simulink model "MultipleAgentsChoice_NoVR"  (R2013b)
settings: Solver=ode45  StartTime=0.0  StopTime=1000  RelTol=1e-4  AbsTol=1e-4
libraries: simulink x24
(part 4 of 5)

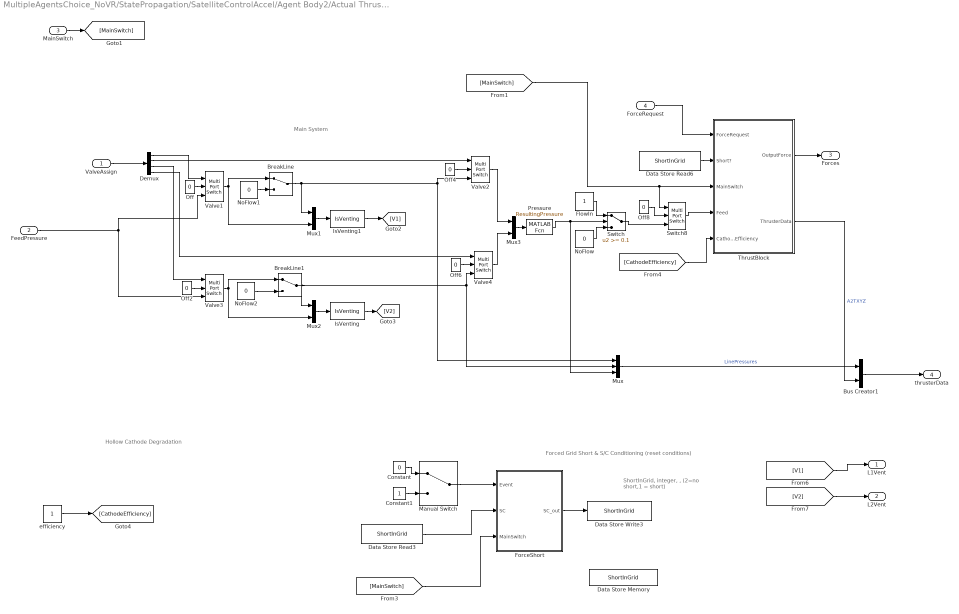
== system MultipleAgentsChoice_NoVR/StatePropagation/SatelliteControlAccel/Agent Body2/Actual Thruster response/XYZthruster/Thruster1 ==
  note: Main System
  note: Hollow Cathode Degradation
  note: ShortInGrid, integer, , (2=no short,1 = short)
  note: Forced Grid Short & S/C Conditioning (reset conditions)
  ValveAssign : Inport
  FeedPressure : Inport  Port=2
  MainSwitch : Inport  Port=3
  ForceRequest : Inport  Port=4
  BreakLine : ManualSwitch
  BreakLine1 : ManualSwitch
  Bus Creator1 : BusCreator  Inputs=2
  Constant : Constant  Value=0
  Constant1 : Constant
  Data Store Memory : DataStoreMemory  DataStoreName=ShortInGrid  ReadBeforeWriteMsg=warning  WriteAfterWriteMsg=warning  WriteAfterReadMsg=warning  InitialValue=2
  Data Store Read3 : DataStoreRead  DataStoreName=ShortInGrid  SampleTime=0
  Data Store Read6 : DataStoreRead  DataStoreName=ShortInGrid  SampleTime=0
  Data Store Write3 : DataStoreWrite  DataStoreName=ShortInGrid
  Demux : Demux
  FlowIn : Constant
  ForceShort : Subsystem
  IsVenting : MATLABFcn  MATLABFcn=IsVenting  OutputDimensions=1
  IsVenting1 : MATLABFcn  MATLABFcn=IsVenting  OutputDimensions=1
  Manual Switch : ManualSwitch
  Mux : Mux  Inputs=3
  Mux1 : Mux  Inputs=2
  Mux2 : Mux  Inputs=2
  Mux3 : Mux  Inputs=2
  NoFlow : Constant  Value=0
  NoFlow1 : Constant  Value=0
  NoFlow2 : Constant  Value=0
  Off{,2,4,6,8} (5 alike) : Constant  Value=0
  Pressure : MATLABFcn  MATLABFcn=ResultingPressure
  Switch : Switch  Threshold=0.1
  Switch8 : MultiPortSwitch  Inputs=2
  ThrustBlock : Subsystem
  Valve{1..4} (4 alike) : MultiPortSwitch  Inputs=2
  efficiency : Constant
  L1Vent : Outport
  L2Vent : Outport  Port=2
  Forces : Outport  Port=3
  thrusterData : Outport  Port=4
  wires:
  [MainSwitch] -> Switch8/1, ThrustBlock/3(MainSwitch)
  Valve4/1 -> Mux3/2
  MainSwitch/1 -> [MainSwitch]
  FeedPressure/1 -> Valve3/3, Valve1/3
  IsVenting/1 -> [V2]
  IsVenting1/1 -> [V1]
  Pressure/1 -> Mux/3, Switch/2
  Mux2/1 -> IsVenting/1
  Mux1/1 -> IsVenting1/1
  Bus Creator1/1 -> thrusterData/1
  ForceRequest/1 -> ThrustBlock/1(ForceRequest)
  [CathodeEfficiency] -> ThrustBlock/5(CathodeEfficiency)
  BreakLine1/1 -> Mux/2, Valve4/3, Mux2/1
  Valve3/1 -> Mux2/2, BreakLine1/1
  NoFlow2/1 -> BreakLine1/2
  Mux/1 -> Bus Creator1/1  "LinePressures"
  Switch/1 -> Switch8/3
  Off8/1 -> Switch8/2
  Off6/1 -> Valve4/2
  Off2/1 -> Valve3/2
  Off4/1 -> Valve2/2
  Off/1 -> Valve1/2
  NoFlow1/1 -> BreakLine/2
  ThrustBlock/1(OutputForce) -> Forces/1
  ThrustBlock/2(ThrusterData) -> Bus Creator1/2  "A2TXYZ"
  Demux/4 -> Valve4/1
  Demux/3 -> Valve3/1
  Demux/2 -> Valve2/1
  Demux/1 -> Valve1/1
  ValveAssign/1 -> Demux/1
  Data Store Read6/1 -> ThrustBlock/2(Short?)
  Switch8/1 -> ThrustBlock/4(Feed)
  NoFlow/1 -> Switch/3
  FlowIn/1 -> Switch/1
  BreakLine/1 -> Mux/1, Valve2/3, Mux1/1
  Mux3/1 -> Pressure/1
  Valve2/1 -> Mux3/1
  Valve1/1 -> Mux1/2, BreakLine/1
  efficiency/1 -> [CathodeEfficiency]
  [MainSwitch] -> ForceShort/3(MainSwitch)
  Data Store Read3/1 -> ForceShort/2(SC)
  Manual Switch/1 -> ForceShort/1(Event)
  Constant1/1 -> Manual Switch/2
  Constant/1 -> Manual Switch/1
  ForceShort/1(SC_out) -> Data Store Write3/1
  [V1] -> L1Vent/1
  [V2] -> L2Vent/1

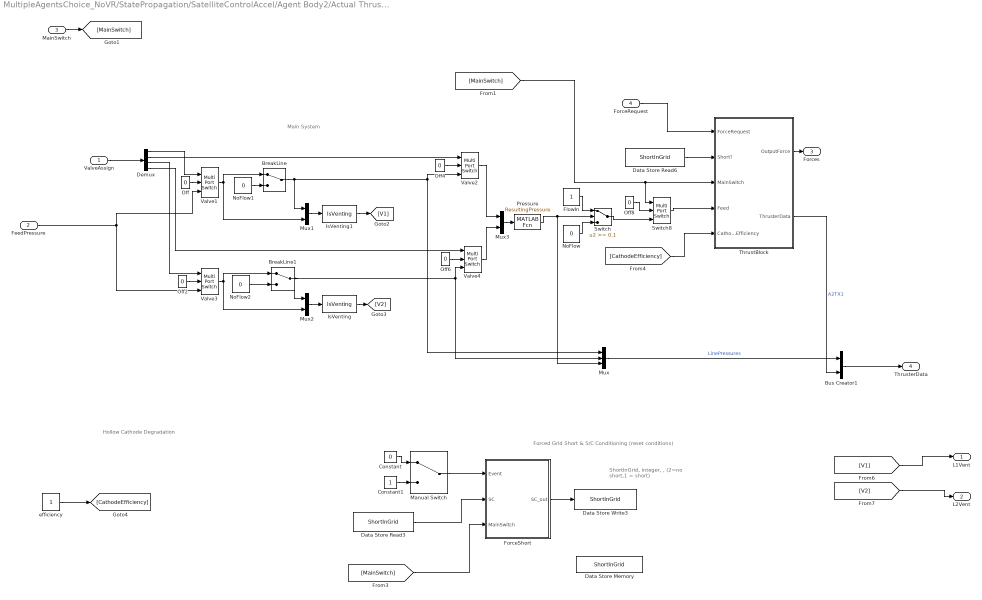
== system MultipleAgentsChoice_NoVR/StatePropagation/SatelliteControlAccel/Agent Body2/Actual Thruster response/Xthruster/Thruster1 ==
  note: Forced Grid Short & S/C Conditioning (reset conditions)
  note: ShortInGrid, integer, , (2=no short,1 = short)
  note: Hollow Cathode Degradation
  note: Main System
  ValveAssign : Inport
  FeedPressure : Inport  Port=2
  MainSwitch : Inport  Port=3
  ForceRequest : Inport  Port=4
  BreakLine : ManualSwitch
  BreakLine1 : ManualSwitch
  Bus Creator1 : BusCreator  Inputs=2
  Constant : Constant  Value=0
  Constant1 : Constant
  Data Store Memory : DataStoreMemory  DataStoreName=ShortInGrid  ReadBeforeWriteMsg=warning  WriteAfterWriteMsg=warning  WriteAfterReadMsg=warning  InitialValue=2
  Data Store Read3 : DataStoreRead  DataStoreName=ShortInGrid  SampleTime=0
  Data Store Read6 : DataStoreRead  DataStoreName=ShortInGrid  SampleTime=0
  Data Store Write3 : DataStoreWrite  DataStoreName=ShortInGrid
  Demux : Demux
  FlowIn : Constant
  ForceShort : Subsystem
  IsVenting : MATLABFcn  MATLABFcn=IsVenting  OutputDimensions=1
  IsVenting1 : MATLABFcn  MATLABFcn=IsVenting  OutputDimensions=1
  Manual Switch : ManualSwitch
  Mux : Mux  Inputs=3
  Mux1 : Mux  Inputs=2
  Mux2 : Mux  Inputs=2
  Mux3 : Mux  Inputs=2
  NoFlow : Constant  Value=0
  NoFlow1 : Constant  Value=0
  NoFlow2 : Constant  Value=0
  Off{,2,4,6,8} (5 alike) : Constant  Value=0
  Pressure : MATLABFcn  MATLABFcn=ResultingPressure
  Switch : Switch  Threshold=0.1
  Switch8 : MultiPortSwitch  Inputs=2
  ThrustBlock : Subsystem
  Valve{1..4} (4 alike) : MultiPortSwitch  Inputs=2
  efficiency : Constant
  L1Vent : Outport
  L2Vent : Outport  Port=2
  Forces : Outport  Port=3
  ThrusterData : Outport  Port=4
  wires:
  ForceShort/1(SC_out) -> Data Store Write3/1
  Constant/1 -> Manual Switch/1
  Constant1/1 -> Manual Switch/2
  Manual Switch/1 -> ForceShort/1(Event)
  Data Store Read3/1 -> ForceShort/2(SC)
  [MainSwitch] -> ForceShort/3(MainSwitch)
  efficiency/1 -> [CathodeEfficiency]
  Valve1/1 -> BreakLine/1, Mux1/2
  Valve2/1 -> Mux3/1
  Mux3/1 -> Pressure/1
  BreakLine/1 -> Mux1/1, Valve2/3, Mux/1
  FlowIn/1 -> Switch/1
  NoFlow/1 -> Switch/3
  Switch8/1 -> ThrustBlock/4(Feed)
  Data Store Read6/1 -> ThrustBlock/2(Short?)
  ValveAssign/1 -> Demux/1
  Demux/1 -> Valve1/1
  Demux/2 -> Valve2/1
  Demux/3 -> Valve3/1
  Demux/4 -> Valve4/1
  ThrustBlock/2(ThrusterData) -> Bus Creator1/2  "A2TX1"
  ThrustBlock/1(OutputForce) -> Forces/1
  NoFlow1/1 -> BreakLine/2
  Off/1 -> Valve1/2
  Off4/1 -> Valve2/2
  Off2/1 -> Valve3/2
  Off6/1 -> Valve4/2
  Off8/1 -> Switch8/2
  Switch/1 -> Switch8/3
  Mux/1 -> Bus Creator1/1  "LinePressures"
  NoFlow2/1 -> BreakLine1/2
  Valve3/1 -> BreakLine1/1, Mux2/2
  BreakLine1/1 -> Mux2/1, Valve4/3, Mux/2
  [CathodeEfficiency] -> ThrustBlock/5(CathodeEfficiency)
  ForceRequest/1 -> ThrustBlock/1(ForceRequest)
  Bus Creator1/1 -> ThrusterData/1
  Mux1/1 -> IsVenting1/1
  Mux2/1 -> IsVenting/1
  Pressure/1 -> Switch/2, Mux/3
  IsVenting1/1 -> [V1]
  IsVenting/1 -> [V2]
  FeedPressure/1 -> Valve1/3, Valve3/3
  MainSwitch/1 -> [MainSwitch]
  Valve4/1 -> Mux3/2
  [MainSwitch] -> ThrustBlock/3(MainSwitch), Switch8/1
  [V1] -> L1Vent/1
  [V2] -> L2Vent/1

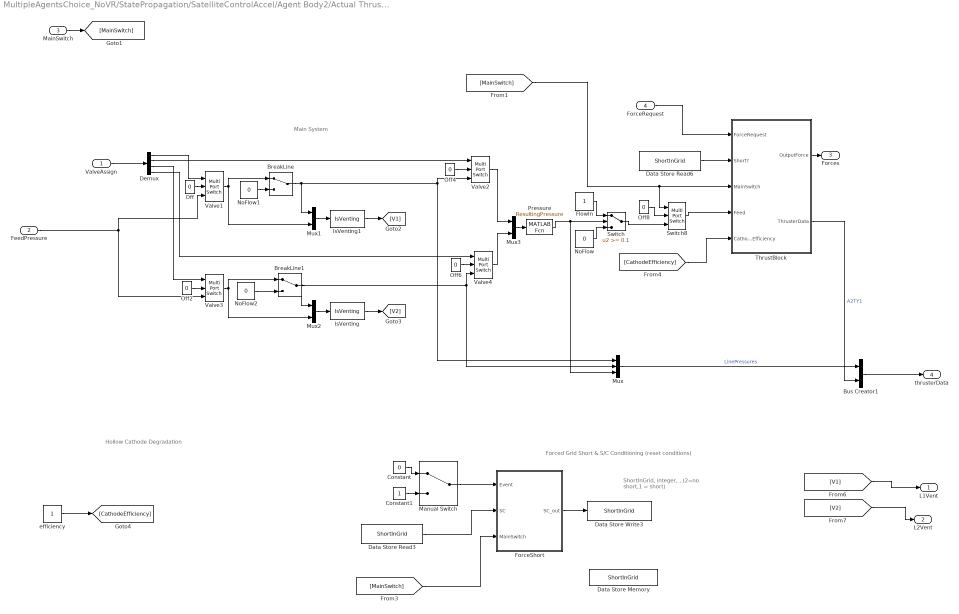
== system MultipleAgentsChoice_NoVR/StatePropagation/SatelliteControlAccel/Agent Body2/Actual Thruster response/Ythruster1/Thruster1 ==
  note: Main System
  note: Hollow Cathode Degradation
  note: ShortInGrid, integer, , (2=no short,1 = short)
  note: Forced Grid Short & S/C Conditioning (reset conditions)
  ValveAssign : Inport
  FeedPressure : Inport  Port=2
  MainSwitch : Inport  Port=3
  ForceRequest : Inport  Port=4
  BreakLine : ManualSwitch
  BreakLine1 : ManualSwitch
  Bus Creator1 : BusCreator  Inputs=2
  Constant : Constant  Value=0
  Constant1 : Constant
  Data Store Memory : DataStoreMemory  DataStoreName=ShortInGrid  ReadBeforeWriteMsg=warning  WriteAfterWriteMsg=warning  WriteAfterReadMsg=warning  InitialValue=2
  Data Store Read3 : DataStoreRead  DataStoreName=ShortInGrid  SampleTime=0
  Data Store Read6 : DataStoreRead  DataStoreName=ShortInGrid  SampleTime=0
  Data Store Write3 : DataStoreWrite  DataStoreName=ShortInGrid
  Demux : Demux
  FlowIn : Constant
  ForceShort : Subsystem
  IsVenting : MATLABFcn  MATLABFcn=IsVenting  OutputDimensions=1
  IsVenting1 : MATLABFcn  MATLABFcn=IsVenting  OutputDimensions=1
  Manual Switch : ManualSwitch
  Mux : Mux  Inputs=3
  Mux1 : Mux  Inputs=2
  Mux2 : Mux  Inputs=2
  Mux3 : Mux  Inputs=2
  NoFlow : Constant  Value=0
  NoFlow1 : Constant  Value=0
  NoFlow2 : Constant  Value=0
  Off{,2,4,6,8} (5 alike) : Constant  Value=0
  Pressure : MATLABFcn  MATLABFcn=ResultingPressure
  Switch : Switch  Threshold=0.1
  Switch8 : MultiPortSwitch  Inputs=2
  ThrustBlock : Subsystem
  Valve{1..4} (4 alike) : MultiPortSwitch  Inputs=2
  efficiency : Constant
  L1Vent : Outport
  L2Vent : Outport  Port=2
  Forces : Outport  Port=3
  thrusterData : Outport  Port=4
  wires:
  [MainSwitch] -> ThrustBlock/3(MainSwitch), Switch8/1
  Valve4/1 -> Mux3/2
  MainSwitch/1 -> [MainSwitch]
  FeedPressure/1 -> Valve3/3, Valve1/3
  IsVenting/1 -> [V2]
  IsVenting1/1 -> [V1]
  Pressure/1 -> Mux/3, Switch/2
  Mux2/1 -> IsVenting/1
  Mux1/1 -> IsVenting1/1
  Bus Creator1/1 -> thrusterData/1
  ForceRequest/1 -> ThrustBlock/1(ForceRequest)
  [CathodeEfficiency] -> ThrustBlock/5(CathodeEfficiency)
  BreakLine1/1 -> Mux/2, Valve4/3, Mux2/1
  Valve3/1 -> Mux2/2, BreakLine1/1
  NoFlow2/1 -> BreakLine1/2
  Mux/1 -> Bus Creator1/1  "LinePressures"
  Switch/1 -> Switch8/3
  Off8/1 -> Switch8/2
  Off6/1 -> Valve4/2
  Off2/1 -> Valve3/2
  Off4/1 -> Valve2/2
  Off/1 -> Valve1/2
  NoFlow1/1 -> BreakLine/2
  ThrustBlock/1(OutputForce) -> Forces/1
  ThrustBlock/2(ThrusterData) -> Bus Creator1/2  "A2TY1"
  Demux/4 -> Valve4/1
  Demux/3 -> Valve3/1
  Demux/2 -> Valve2/1
  Demux/1 -> Valve1/1
  ValveAssign/1 -> Demux/1
  Data Store Read6/1 -> ThrustBlock/2(Short?)
  Switch8/1 -> ThrustBlock/4(Feed)
  NoFlow/1 -> Switch/3
  FlowIn/1 -> Switch/1
  BreakLine/1 -> Mux/1, Valve2/3, Mux1/1
  Mux3/1 -> Pressure/1
  Valve2/1 -> Mux3/1
  Valve1/1 -> Mux1/2, BreakLine/1
  efficiency/1 -> [CathodeEfficiency]
  [MainSwitch] -> ForceShort/3(MainSwitch)
  Data Store Read3/1 -> ForceShort/2(SC)
  Manual Switch/1 -> ForceShort/1(Event)
  Constant1/1 -> Manual Switch/2
  Constant/1 -> Manual Switch/1
  ForceShort/1(SC_out) -> Data Store Write3/1
  [V1] -> L1Vent/1
  [V2] -> L2Vent/1

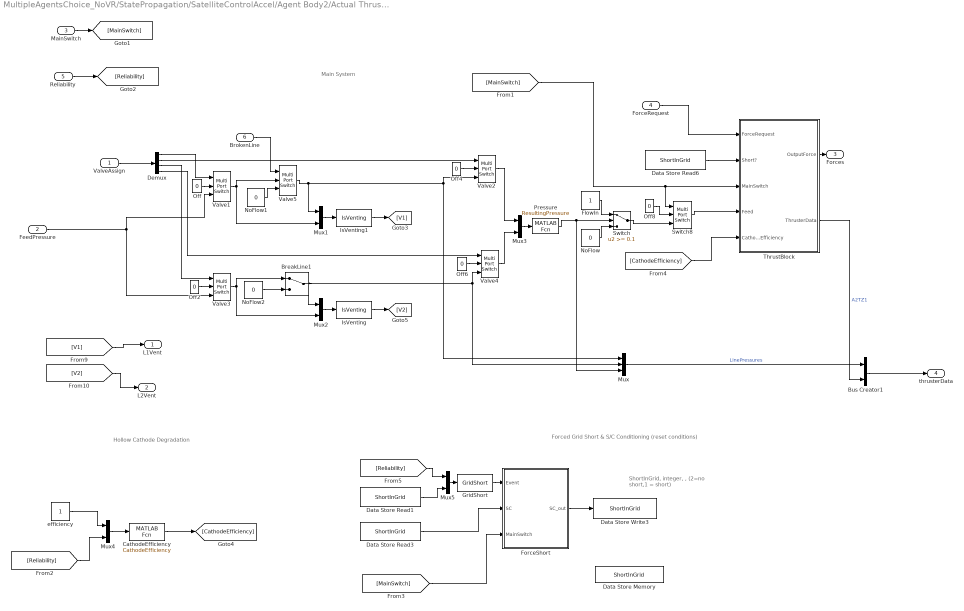
== system MultipleAgentsChoice_NoVR/StatePropagation/SatelliteControlAccel/Agent Body2/Actual Thruster response/Zthruster1/Thruster1 ==
  note: Forced Grid Short & S/C Conditioning (reset conditions)
  note: ShortInGrid, integer, , (2=no short,1 = short)
  note: Hollow Cathode Degradation
  note: Main System
  ValveAssign : Inport
  FeedPressure : Inport  Port=2
  MainSwitch : Inport  Port=3
  ForceRequest : Inport  Port=4
  Reliability : Inport  Port=5
  BrokenLine : Inport  Port=6
  BreakLine1 : ManualSwitch
  Bus Creator1 : BusCreator  Inputs=2
  CathodeEfficiency : MATLABFcn  MATLABFcn=CathodeEfficiency  OutputDimensions=1
  Data Store Memory : DataStoreMemory  DataStoreName=ShortInGrid  ReadBeforeWriteMsg=warning  WriteAfterWriteMsg=warning  WriteAfterReadMsg=warning  InitialValue=2
  Data Store Read1 : DataStoreRead  DataStoreName=ShortInGrid  SampleTime=0
  Data Store Read3 : DataStoreRead  DataStoreName=ShortInGrid  SampleTime=0
  Data Store Read6 : DataStoreRead  DataStoreName=ShortInGrid  SampleTime=0
  Data Store Write3 : DataStoreWrite  DataStoreName=ShortInGrid
  Demux : Demux
  FlowIn : Constant
  ForceShort : Subsystem
  GridShort : MATLABFcn  MATLABFcn=GridShort  OutputDimensions=1
  IsVenting : MATLABFcn  MATLABFcn=IsVenting  OutputDimensions=1
  IsVenting1 : MATLABFcn  MATLABFcn=IsVenting  OutputDimensions=1
  Mux : Mux  Inputs=3
  Mux{1..5} (5 alike) : Mux  Inputs=2
  NoFlow : Constant  Value=0
  NoFlow1 : Constant  Value=0
  NoFlow2 : Constant  Value=0
  Off{,2,4,6,8} (5 alike) : Constant  Value=0
  Pressure : MATLABFcn  MATLABFcn=ResultingPressure
  Switch : Switch  Threshold=0.1
  Switch8 : MultiPortSwitch  Inputs=2
  ThrustBlock : Subsystem
  Valve{1..5} (5 alike) : MultiPortSwitch  Inputs=2
  efficiency : Constant
  L1Vent : Outport
  L2Vent : Outport  Port=2
  Forces : Outport  Port=3
  thrusterData : Outport  Port=4
  wires:
  ForceShort/1(SC_out) -> Data Store Write3/1
  GridShort/1 -> ForceShort/1(Event)
  Data Store Read3/1 -> ForceShort/2(SC)
  [MainSwitch] -> ForceShort/3(MainSwitch)
  Valve1/1 -> Mux1/2, Valve5/2
  Valve2/1 -> Mux3/1
  Mux3/1 -> Pressure/1
  Valve5/1 -> Mux1/1, Valve2/3, Mux/1
  FlowIn/1 -> Switch/1
  NoFlow/1 -> Switch/3
  Switch8/1 -> ThrustBlock/4(Feed)
  Data Store Read6/1 -> ThrustBlock/2(Short?)
  ValveAssign/1 -> Demux/1
  Demux/1 -> Valve1/1
  Demux/2 -> Valve2/1
  Demux/3 -> Valve3/1
  Demux/4 -> Valve4/1
  ThrustBlock/2(ThrusterData) -> Bus Creator1/2  "A2TZ1"
  ThrustBlock/1(OutputForce) -> Forces/1
  NoFlow1/1 -> Valve5/3
  Off/1 -> Valve1/2
  Off4/1 -> Valve2/2
  Off2/1 -> Valve3/2
  Off6/1 -> Valve4/2
  Off8/1 -> Switch8/2
  Switch/1 -> Switch8/3
  Mux/1 -> Bus Creator1/1  "LinePressures"
  NoFlow2/1 -> BreakLine1/2
  Valve3/1 -> BreakLine1/1, Mux2/2
  BreakLine1/1 -> Mux2/1, Valve4/3, Mux/2
  [CathodeEfficiency] -> ThrustBlock/5(CathodeEfficiency)
  ForceRequest/1 -> ThrustBlock/1(ForceRequest)
  Bus Creator1/1 -> thrusterData/1
  Mux1/1 -> IsVenting1/1
  Mux2/1 -> IsVenting/1
  Pressure/1 -> Switch/2, Mux/3
  IsVenting1/1 -> [V1]
  IsVenting/1 -> [V2]
  FeedPressure/1 -> Valve1/3, Valve3/3
  MainSwitch/1 -> [MainSwitch]
  Valve4/1 -> Mux3/2
  [MainSwitch] -> ThrustBlock/3(MainSwitch), Switch8/1
  Reliability/1 -> [Reliability]
  efficiency/1 -> Mux4/1
  [Reliability] -> Mux4/2
  Mux4/1 -> CathodeEfficiency/1
  CathodeEfficiency/1 -> [CathodeEfficiency]
  Mux5/1 -> GridShort/1
  Data Store Read1/1 -> Mux5/2
  [Reliability] -> Mux5/1
  BrokenLine/1 -> Valve5/1
  [V1] -> L1Vent/1
  [V2] -> L2Vent/1

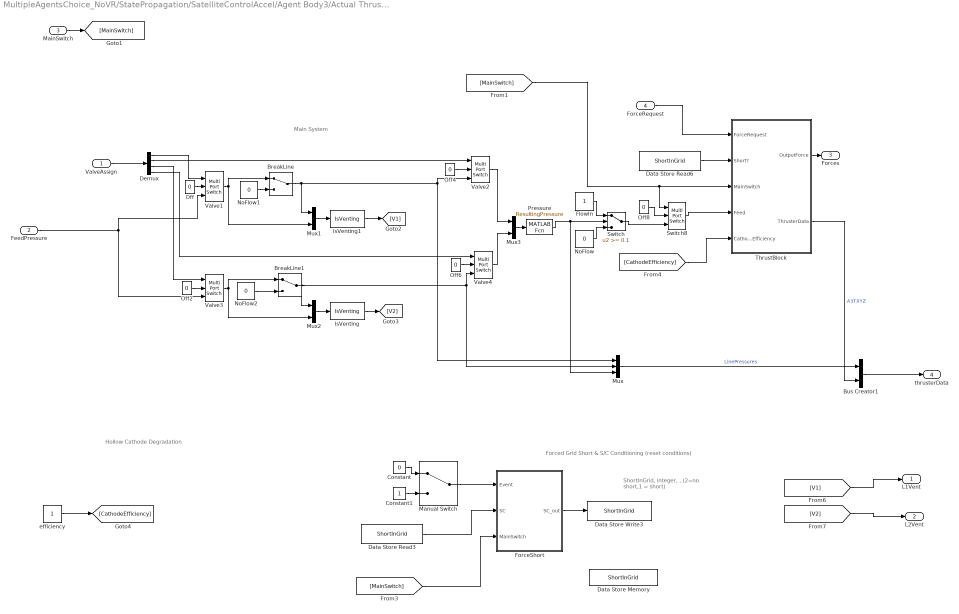
== system MultipleAgentsChoice_NoVR/StatePropagation/SatelliteControlAccel/Agent Body3/Actual Thruster response/XYZthruster/Thruster1 ==
  note: Main System
  note: Hollow Cathode Degradation
  note: ShortInGrid, integer, , (2=no short,1 = short)
  note: Forced Grid Short & S/C Conditioning (reset conditions)
  ValveAssign : Inport
  FeedPressure : Inport  Port=2
  MainSwitch : Inport  Port=3
  ForceRequest : Inport  Port=4
  BreakLine : ManualSwitch
  BreakLine1 : ManualSwitch
  Bus Creator1 : BusCreator  Inputs=2
  Constant : Constant  Value=0
  Constant1 : Constant
  Data Store Memory : DataStoreMemory  DataStoreName=ShortInGrid  ReadBeforeWriteMsg=warning  WriteAfterWriteMsg=warning  WriteAfterReadMsg=warning  InitialValue=2
  Data Store Read3 : DataStoreRead  DataStoreName=ShortInGrid  SampleTime=0
  Data Store Read6 : DataStoreRead  DataStoreName=ShortInGrid  SampleTime=0
  Data Store Write3 : DataStoreWrite  DataStoreName=ShortInGrid
  Demux : Demux
  FlowIn : Constant
  ForceShort : Subsystem
  IsVenting : MATLABFcn  MATLABFcn=IsVenting  OutputDimensions=1
  IsVenting1 : MATLABFcn  MATLABFcn=IsVenting  OutputDimensions=1
  Manual Switch : ManualSwitch
  Mux : Mux  Inputs=3
  Mux1 : Mux  Inputs=2
  Mux2 : Mux  Inputs=2
  Mux3 : Mux  Inputs=2
  NoFlow : Constant  Value=0
  NoFlow1 : Constant  Value=0
  NoFlow2 : Constant  Value=0
  Off{,2,4,6,8} (5 alike) : Constant  Value=0
  Pressure : MATLABFcn  MATLABFcn=ResultingPressure
  Switch : Switch  Threshold=0.1
  Switch8 : MultiPortSwitch  Inputs=2
  ThrustBlock : Subsystem
  Valve{1..4} (4 alike) : MultiPortSwitch  Inputs=2
  efficiency : Constant
  L1Vent : Outport
  L2Vent : Outport  Port=2
  Forces : Outport  Port=3
  thrusterData : Outport  Port=4
  wires:
  [MainSwitch] -> Switch8/1, ThrustBlock/3(MainSwitch)
  Valve4/1 -> Mux3/2
  MainSwitch/1 -> [MainSwitch]
  FeedPressure/1 -> Valve3/3, Valve1/3
  IsVenting/1 -> [V2]
  IsVenting1/1 -> [V1]
  Pressure/1 -> Mux/3, Switch/2
  Mux2/1 -> IsVenting/1
  Mux1/1 -> IsVenting1/1
  Bus Creator1/1 -> thrusterData/1
  ForceRequest/1 -> ThrustBlock/1(ForceRequest)
  [CathodeEfficiency] -> ThrustBlock/5(CathodeEfficiency)
  BreakLine1/1 -> Mux/2, Valve4/3, Mux2/1
  Valve3/1 -> Mux2/2, BreakLine1/1
  NoFlow2/1 -> BreakLine1/2
  Mux/1 -> Bus Creator1/1  "LinePressures"
  Switch/1 -> Switch8/3
  Off8/1 -> Switch8/2
  Off6/1 -> Valve4/2
  Off2/1 -> Valve3/2
  Off4/1 -> Valve2/2
  Off/1 -> Valve1/2
  NoFlow1/1 -> BreakLine/2
  ThrustBlock/1(OutputForce) -> Forces/1
  ThrustBlock/2(ThrusterData) -> Bus Creator1/2  "A3TXYZ"
  Demux/4 -> Valve4/1
  Demux/3 -> Valve3/1
  Demux/2 -> Valve2/1
  Demux/1 -> Valve1/1
  ValveAssign/1 -> Demux/1
  Data Store Read6/1 -> ThrustBlock/2(Short?)
  Switch8/1 -> ThrustBlock/4(Feed)
  NoFlow/1 -> Switch/3
  FlowIn/1 -> Switch/1
  BreakLine/1 -> Mux/1, Valve2/3, Mux1/1
  Mux3/1 -> Pressure/1
  Valve2/1 -> Mux3/1
  Valve1/1 -> Mux1/2, BreakLine/1
  efficiency/1 -> [CathodeEfficiency]
  [MainSwitch] -> ForceShort/3(MainSwitch)
  Data Store Read3/1 -> ForceShort/2(SC)
  Manual Switch/1 -> ForceShort/1(Event)
  Constant1/1 -> Manual Switch/2
  Constant/1 -> Manual Switch/1
  ForceShort/1(SC_out) -> Data Store Write3/1
  [V1] -> L1Vent/1
  [V2] -> L2Vent/1

== system MultipleAgentsChoice_NoVR/StatePropagation/SatelliteControlAccel/Agent Body3/Actual Thruster response/Xthruster/Thruster1 ==
  note: Forced Grid Short & S/C Conditioning (reset conditions)
  note: ShortInGrid, integer, , (2=no short,1 = short)
  note: Hollow Cathode Degradation
  note: Main System
  ValveAssign : Inport
  FeedPressure : Inport  Port=2
  MainSwitch : Inport  Port=3
  ForceRequest : Inport  Port=4
  BreakLine : ManualSwitch
  BreakLine1 : ManualSwitch
  Bus Creator1 : BusCreator  Inputs=2
  Constant : Constant  Value=0
  Constant1 : Constant
  Data Store Memory : DataStoreMemory  DataStoreName=ShortInGrid  ReadBeforeWriteMsg=warning  WriteAfterWriteMsg=warning  WriteAfterReadMsg=warning  InitialValue=2
  Data Store Read3 : DataStoreRead  DataStoreName=ShortInGrid  SampleTime=0
  Data Store Read6 : DataStoreRead  DataStoreName=ShortInGrid  SampleTime=0
  Data Store Write3 : DataStoreWrite  DataStoreName=ShortInGrid
  Demux : Demux
  FlowIn : Constant
  ForceShort : Subsystem
  IsVenting : MATLABFcn  MATLABFcn=IsVenting  OutputDimensions=1
  IsVenting1 : MATLABFcn  MATLABFcn=IsVenting  OutputDimensions=1
  Manual Switch : ManualSwitch
  Mux : Mux  Inputs=3
  Mux1 : Mux  Inputs=2
  Mux2 : Mux  Inputs=2
  Mux3 : Mux  Inputs=2
  NoFlow : Constant  Value=0
  NoFlow1 : Constant  Value=0
  NoFlow2 : Constant  Value=0
  Off{,2,4,6,8} (5 alike) : Constant  Value=0
  Pressure : MATLABFcn  MATLABFcn=ResultingPressure
  Switch : Switch  Threshold=0.1
  Switch8 : MultiPortSwitch  Inputs=2
  ThrustBlock : Subsystem
  Valve{1..4} (4 alike) : MultiPortSwitch  Inputs=2
  efficiency : Constant
  L1Vent : Outport
  L2Vent : Outport  Port=2
  Forces : Outport  Port=3
  ThrusterData : Outport  Port=4
  wires:
  ForceShort/1(SC_out) -> Data Store Write3/1
  Constant/1 -> Manual Switch/1
  Constant1/1 -> Manual Switch/2
  Manual Switch/1 -> ForceShort/1(Event)
  Data Store Read3/1 -> ForceShort/2(SC)
  [MainSwitch] -> ForceShort/3(MainSwitch)
  efficiency/1 -> [CathodeEfficiency]
  Valve1/1 -> BreakLine/1, Mux1/2
  Valve2/1 -> Mux3/1
  Mux3/1 -> Pressure/1
  BreakLine/1 -> Mux1/1, Valve2/3, Mux/1
  FlowIn/1 -> Switch/1
  NoFlow/1 -> Switch/3
  Switch8/1 -> ThrustBlock/4(Feed)
  Data Store Read6/1 -> ThrustBlock/2(Short?)
  ValveAssign/1 -> Demux/1
  Demux/1 -> Valve1/1
  Demux/2 -> Valve2/1
  Demux/3 -> Valve3/1
  Demux/4 -> Valve4/1
  ThrustBlock/2(ThrusterData) -> Bus Creator1/2  "A3TX1"
  ThrustBlock/1(OutputForce) -> Forces/1
  NoFlow1/1 -> BreakLine/2
  Off/1 -> Valve1/2
  Off4/1 -> Valve2/2
  Off2/1 -> Valve3/2
  Off6/1 -> Valve4/2
  Off8/1 -> Switch8/2
  Switch/1 -> Switch8/3
  Mux/1 -> Bus Creator1/1  "LinePressures"
  NoFlow2/1 -> BreakLine1/2
  Valve3/1 -> BreakLine1/1, Mux2/2
  BreakLine1/1 -> Mux2/1, Valve4/3, Mux/2
  [CathodeEfficiency] -> ThrustBlock/5(CathodeEfficiency)
  ForceRequest/1 -> ThrustBlock/1(ForceRequest)
  Bus Creator1/1 -> ThrusterData/1
  Mux1/1 -> IsVenting1/1
  Mux2/1 -> IsVenting/1
  Pressure/1 -> Switch/2, Mux/3
  IsVenting1/1 -> [V1]
  IsVenting/1 -> [V2]
  FeedPressure/1 -> Valve1/3, Valve3/3
  MainSwitch/1 -> [MainSwitch]
  Valve4/1 -> Mux3/2
  [MainSwitch] -> ThrustBlock/3(MainSwitch), Switch8/1
  [V1] -> L1Vent/1
  [V2] -> L2Vent/1

== system MultipleAgentsChoice_NoVR/StatePropagation/SatelliteControlAccel/Agent Body3/Actual Thruster response/Ythruster1/Thruster1 ==
  note: Main System
  note: Hollow Cathode Degradation
  note: ShortInGrid, integer, , (2=no short,1 = short)
  note: Forced Grid Short & S/C Conditioning (reset conditions)
  ValveAssign : Inport
  FeedPressure : Inport  Port=2
  MainSwitch : Inport  Port=3
  ForceRequest : Inport  Port=4
  BreakLine : ManualSwitch
  BreakLine1 : ManualSwitch
  Bus Creator1 : BusCreator  Inputs=2
  Constant : Constant  Value=0
  Constant1 : Constant
  Data Store Memory : DataStoreMemory  DataStoreName=ShortInGrid  ReadBeforeWriteMsg=warning  WriteAfterWriteMsg=warning  WriteAfterReadMsg=warning  InitialValue=2
  Data Store Read3 : DataStoreRead  DataStoreName=ShortInGrid  SampleTime=0
  Data Store Read6 : DataStoreRead  DataStoreName=ShortInGrid  SampleTime=0
  Data Store Write3 : DataStoreWrite  DataStoreName=ShortInGrid
  Demux : Demux
  FlowIn : Constant
  ForceShort : Subsystem
  IsVenting : MATLABFcn  MATLABFcn=IsVenting  OutputDimensions=1
  IsVenting1 : MATLABFcn  MATLABFcn=IsVenting  OutputDimensions=1
  Manual Switch : ManualSwitch
  Mux : Mux  Inputs=3
  Mux1 : Mux  Inputs=2
  Mux2 : Mux  Inputs=2
  Mux3 : Mux  Inputs=2
  NoFlow : Constant  Value=0
  NoFlow1 : Constant  Value=0
  NoFlow2 : Constant  Value=0
  Off{,2,4,6,8} (5 alike) : Constant  Value=0
  Pressure : MATLABFcn  MATLABFcn=ResultingPressure
  Switch : Switch  Threshold=0.1
  Switch8 : MultiPortSwitch  Inputs=2
  ThrustBlock : Subsystem
  Valve{1..4} (4 alike) : MultiPortSwitch  Inputs=2
  efficiency : Constant
  L1Vent : Outport
  L2Vent : Outport  Port=2
  Forces : Outport  Port=3
  thrusterData : Outport  Port=4
  wires:
  [MainSwitch] -> ThrustBlock/3(MainSwitch), Switch8/1
  Valve4/1 -> Mux3/2
  MainSwitch/1 -> [MainSwitch]
  FeedPressure/1 -> Valve3/3, Valve1/3
  IsVenting/1 -> [V2]
  IsVenting1/1 -> [V1]
  Pressure/1 -> Mux/3, Switch/2
  Mux2/1 -> IsVenting/1
  Mux1/1 -> IsVenting1/1
  Bus Creator1/1 -> thrusterData/1
  ForceRequest/1 -> ThrustBlock/1(ForceRequest)
  [CathodeEfficiency] -> ThrustBlock/5(CathodeEfficiency)
  BreakLine1/1 -> Mux/2, Valve4/3, Mux2/1
  Valve3/1 -> Mux2/2, BreakLine1/1
  NoFlow2/1 -> BreakLine1/2
  Mux/1 -> Bus Creator1/1  "LinePressures"
  Switch/1 -> Switch8/3
  Off8/1 -> Switch8/2
  Off6/1 -> Valve4/2
  Off2/1 -> Valve3/2
  Off4/1 -> Valve2/2
  Off/1 -> Valve1/2
  NoFlow1/1 -> BreakLine/2
  ThrustBlock/1(OutputForce) -> Forces/1
  ThrustBlock/2(ThrusterData) -> Bus Creator1/2  "A3TY1"
  Demux/4 -> Valve4/1
  Demux/3 -> Valve3/1
  Demux/2 -> Valve2/1
  Demux/1 -> Valve1/1
  ValveAssign/1 -> Demux/1
  Data Store Read6/1 -> ThrustBlock/2(Short?)
  Switch8/1 -> ThrustBlock/4(Feed)
  NoFlow/1 -> Switch/3
  FlowIn/1 -> Switch/1
  BreakLine/1 -> Mux/1, Valve2/3, Mux1/1
  Mux3/1 -> Pressure/1
  Valve2/1 -> Mux3/1
  Valve1/1 -> Mux1/2, BreakLine/1
  efficiency/1 -> [CathodeEfficiency]
  [MainSwitch] -> ForceShort/3(MainSwitch)
  Data Store Read3/1 -> ForceShort/2(SC)
  Manual Switch/1 -> ForceShort/1(Event)
  Constant1/1 -> Manual Switch/2
  Constant/1 -> Manual Switch/1
  ForceShort/1(SC_out) -> Data Store Write3/1
  [V1] -> L1Vent/1
  [V2] -> L2Vent/1

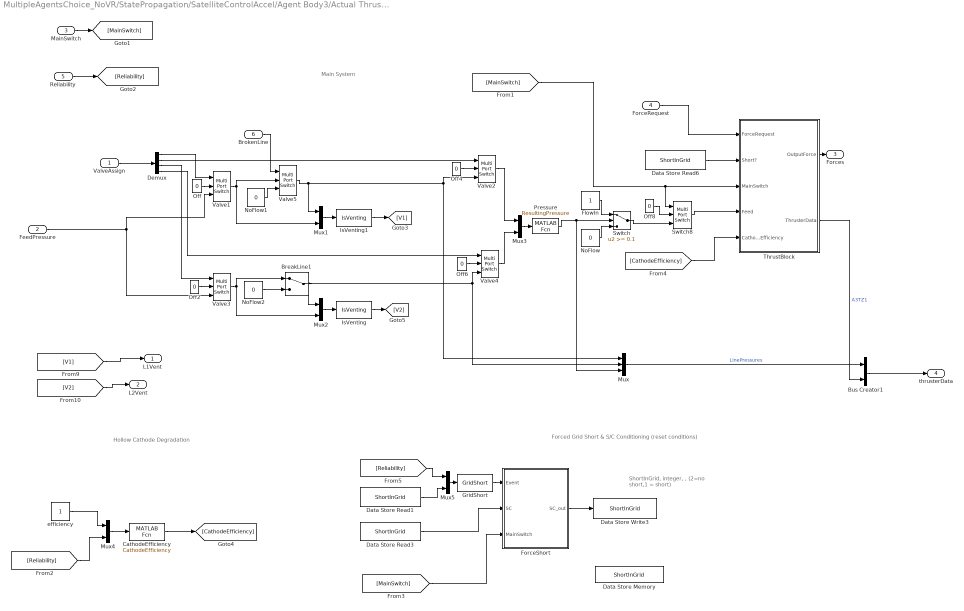
== system MultipleAgentsChoice_NoVR/StatePropagation/SatelliteControlAccel/Agent Body3/Actual Thruster response/Zthruster1/Thruster1 ==
  note: Forced Grid Short & S/C Conditioning (reset conditions)
  note: ShortInGrid, integer, , (2=no short,1 = short)
  note: Hollow Cathode Degradation
  note: Main System
  ValveAssign : Inport
  FeedPressure : Inport  Port=2
  MainSwitch : Inport  Port=3
  ForceRequest : Inport  Port=4
  Reliability : Inport  Port=5
  BrokenLine : Inport  Port=6
  BreakLine1 : ManualSwitch
  Bus Creator1 : BusCreator  Inputs=2
  CathodeEfficiency : MATLABFcn  MATLABFcn=CathodeEfficiency  OutputDimensions=1
  Data Store Memory : DataStoreMemory  DataStoreName=ShortInGrid  ReadBeforeWriteMsg=warning  WriteAfterWriteMsg=warning  WriteAfterReadMsg=warning  InitialValue=2
  Data Store Read1 : DataStoreRead  DataStoreName=ShortInGrid  SampleTime=0
  Data Store Read3 : DataStoreRead  DataStoreName=ShortInGrid  SampleTime=0
  Data Store Read6 : DataStoreRead  DataStoreName=ShortInGrid  SampleTime=0
  Data Store Write3 : DataStoreWrite  DataStoreName=ShortInGrid
  Demux : Demux
  FlowIn : Constant
  ForceShort : Subsystem
  GridShort : MATLABFcn  MATLABFcn=GridShort  OutputDimensions=1
  IsVenting : MATLABFcn  MATLABFcn=IsVenting  OutputDimensions=1
  IsVenting1 : MATLABFcn  MATLABFcn=IsVenting  OutputDimensions=1
  Mux : Mux  Inputs=3
  Mux{1..5} (5 alike) : Mux  Inputs=2
  NoFlow : Constant  Value=0
  NoFlow1 : Constant  Value=0
  NoFlow2 : Constant  Value=0
  Off{,2,4,6,8} (5 alike) : Constant  Value=0
  Pressure : MATLABFcn  MATLABFcn=ResultingPressure
  Switch : Switch  Threshold=0.1
  Switch8 : MultiPortSwitch  Inputs=2
  ThrustBlock : Subsystem
  Valve{1..5} (5 alike) : MultiPortSwitch  Inputs=2
  efficiency : Constant
  L1Vent : Outport
  L2Vent : Outport  Port=2
  Forces : Outport  Port=3
  thrusterData : Outport  Port=4
  wires:
  ForceShort/1(SC_out) -> Data Store Write3/1
  GridShort/1 -> ForceShort/1(Event)
  Data Store Read3/1 -> ForceShort/2(SC)
  [MainSwitch] -> ForceShort/3(MainSwitch)
  Valve1/1 -> Mux1/2, Valve5/2
  Valve2/1 -> Mux3/1
  Mux3/1 -> Pressure/1
  Valve5/1 -> Mux1/1, Valve2/3, Mux/1
  FlowIn/1 -> Switch/1
  NoFlow/1 -> Switch/3
  Switch8/1 -> ThrustBlock/4(Feed)
  Data Store Read6/1 -> ThrustBlock/2(Short?)
  ValveAssign/1 -> Demux/1
  Demux/1 -> Valve1/1
  Demux/2 -> Valve2/1
  Demux/3 -> Valve3/1
  Demux/4 -> Valve4/1
  ThrustBlock/2(ThrusterData) -> Bus Creator1/2  "A3TZ1"
  ThrustBlock/1(OutputForce) -> Forces/1
  NoFlow1/1 -> Valve5/3
  Off/1 -> Valve1/2
  Off4/1 -> Valve2/2
  Off2/1 -> Valve3/2
  Off6/1 -> Valve4/2
  Off8/1 -> Switch8/2
  Switch/1 -> Switch8/3
  Mux/1 -> Bus Creator1/1  "LinePressures"
  NoFlow2/1 -> BreakLine1/2
  Valve3/1 -> BreakLine1/1, Mux2/2
  BreakLine1/1 -> Mux2/1, Valve4/3, Mux/2
  [CathodeEfficiency] -> ThrustBlock/5(CathodeEfficiency)
  ForceRequest/1 -> ThrustBlock/1(ForceRequest)
  Bus Creator1/1 -> thrusterData/1
  Mux1/1 -> IsVenting1/1
  Mux2/1 -> IsVenting/1
  Pressure/1 -> Switch/2, Mux/3
  IsVenting1/1 -> [V1]
  IsVenting/1 -> [V2]
  FeedPressure/1 -> Valve1/3, Valve3/3
  MainSwitch/1 -> [MainSwitch]
  Valve4/1 -> Mux3/2
  [MainSwitch] -> ThrustBlock/3(MainSwitch), Switch8/1
  Reliability/1 -> [Reliability]
  efficiency/1 -> Mux4/1
  [Reliability] -> Mux4/2
  Mux4/1 -> CathodeEfficiency/1
  CathodeEfficiency/1 -> [CathodeEfficiency]
  Mux5/1 -> GridShort/1
  Data Store Read1/1 -> Mux5/2
  [Reliability] -> Mux5/1
  BrokenLine/1 -> Valve5/1
  [V1] -> L1Vent/1
  [V2] -> L2Vent/1

== system MultipleAgentsChoice_NoVR/StatePropagation/SatelliteControlAccel/Agent Body1/Actual Thruster response/XYZthruster/Thruster1/ForceShort ==
  note: Detect event and introduce short, otherwise pass through current result of short status
  Event : Inport
  SC : Inport  Port=2
  MainSwitch : Inport  Port=3
  Constant : Constant
  Data Type Conversion : DataTypeConversion
  Detect Increase : simulink/Logic and Bit Operations/Detect Increase  vinit=0  InputProcessing=Inherited  OutDataTypeStr=uint8
  Multiport Switch : MultiPortSwitch  DataPortOrder=Zero-based contiguous  Inputs=2  zeroidx=on
  S/C Conditioning : Subsystem
  SC_out : Outport
  wires:
  Event/1 -> Detect Increase/1
  Detect Increase/1 -> Data Type Conversion/1
  S/C Conditioning/1(Short?) -> SC_out/1
  MainSwitch/1 -> S/C Conditioning/2(MainSwitch)
  Data Type Conversion/1 -> Multiport Switch/1
  SC/1 -> Multiport Switch/2
  Constant/1 -> Multiport Switch/3
  Multiport Switch/1 -> S/C Conditioning/1(SC)

== system MultipleAgentsChoice_NoVR/StatePropagation/SatelliteControlAccel/Agent Body1/Actual Thruster response/XYZthruster/Thruster1/ThrustBlock ==
  ForceRequest : Inport
  Short? : Inport  Port=2
  MainSwitch : Inport  Port=3
  Feed : Inport  Port=4
  CathodeEfficiency : Inport  Port=5
  ActiveThruster (logical) : Subsystem
  Bus Creator : BusCreator  Inputs=2
  Product : Product  RndMeth=Zero
  Product1 : Product  RndMeth=Zero
  Voltage/Current : Subsystem
  OutputForce : Outport
  ThrusterData : Outport  Port=2
  wires:
  MainSwitch/1 -> ActiveThruster (logical)/2(ThrusterOn?), Voltage/Current/2(MainSwitch)
  Short?/1 -> ActiveThruster (logical)/1(Short?), Voltage/Current/1(Short?)
  Feed/1 -> Voltage/Current/3(Feed?), ActiveThruster (logical)/3(Feed?)
  Voltage/Current/1(Voltage) -> Bus Creator/1  "voltage"
  Voltage/Current/2(Current) -> Bus Creator/2  "current"
  Bus Creator/1 -> ThrusterData/1
  ActiveThruster (logical)/1(Active) -> Product/1
  ForceRequest/1 -> [ForceRequest]
  CathodeEfficiency/1 -> [CathodeEfficiency]
  Product1/1 -> OutputForce/1
  [ForceRequest] -> Product/2
  Product/1 -> Product1/1
  [CathodeEfficiency] -> Product1/2

== system MultipleAgentsChoice_NoVR/StatePropagation/SatelliteControlAccel/Agent Body1/Actual Thruster response/Xthruster/Thruster1/ForceShort ==
  note: Detect event and introduce short, otherwise pass through current result of short status
  Event : Inport
  SC : Inport  Port=2
  MainSwitch : Inport  Port=3
  Constant : Constant
  Data Type Conversion : DataTypeConversion
  Detect Increase : simulink/Logic and Bit Operations/Detect Increase  vinit=0  InputProcessing=Inherited  OutDataTypeStr=uint8
  Multiport Switch : MultiPortSwitch  DataPortOrder=Zero-based contiguous  Inputs=2  zeroidx=on
  S/C Conditioning : Subsystem
  SC_out : Outport
  wires:
  Multiport Switch/1 -> S/C Conditioning/1(SC)
  Constant/1 -> Multiport Switch/3
  SC/1 -> Multiport Switch/2
  Data Type Conversion/1 -> Multiport Switch/1
  MainSwitch/1 -> S/C Conditioning/2(MainSwitch)
  S/C Conditioning/1(Short?) -> SC_out/1
  Detect Increase/1 -> Data Type Conversion/1
  Event/1 -> Detect Increase/1

== system MultipleAgentsChoice_NoVR/StatePropagation/SatelliteControlAccel/Agent Body1/Actual Thruster response/Xthruster/Thruster1/ThrustBlock ==
  ForceRequest : Inport
  Short? : Inport  Port=2
  MainSwitch : Inport  Port=3
  Feed : Inport  Port=4
  CathodeEfficiency : Inport  Port=5
  ActiveThruster (logical) : Subsystem
  Bus Creator : BusCreator  Inputs=2
  Product : Product  RndMeth=Zero
  Product1 : Product  RndMeth=Zero
  Voltage/Current : Subsystem
  OutputForce : Outport
  ThrusterData : Outport  Port=2
  wires:
  [CathodeEfficiency] -> Product1/2
  Product/1 -> Product1/1
  [ForceRequest] -> Product/2
  CathodeEfficiency/1 -> [CathodeEfficiency]
  ForceRequest/1 -> [ForceRequest]
  ActiveThruster (logical)/1(Active) -> Product/1
  Bus Creator/1 -> ThrusterData/1
  Voltage/Current/2(Current) -> Bus Creator/2  "current"
  Voltage/Current/1(Voltage) -> Bus Creator/1  "voltage"
  Feed/1 -> ActiveThruster (logical)/3(Feed?), Voltage/Current/3(Feed?)
  Short?/1 -> Voltage/Current/1(Short?), ActiveThruster (logical)/1(Short?)
  MainSwitch/1 -> Voltage/Current/2(MainSwitch), ActiveThruster (logical)/2(ThrusterOn?)
  Product1/1 -> OutputForce/1

== system MultipleAgentsChoice_NoVR/StatePropagation/SatelliteControlAccel/Agent Body1/Actual Thruster response/Ythruster1/Thruster1/ForceShort ==
  note: Detect event and introduce short, otherwise pass through current result of short status
  Event : Inport
  SC : Inport  Port=2
  MainSwitch : Inport  Port=3
  Constant : Constant
  Data Type Conversion : DataTypeConversion
  Detect Increase : simulink/Logic and Bit Operations/Detect Increase  vinit=0  InputProcessing=Inherited  OutDataTypeStr=uint8
  Multiport Switch : MultiPortSwitch  DataPortOrder=Zero-based contiguous  Inputs=2  zeroidx=on
  S/C Conditioning : Subsystem
  SC_out : Outport
  wires:
  Event/1 -> Detect Increase/1
  Detect Increase/1 -> Data Type Conversion/1
  S/C Conditioning/1(Short?) -> SC_out/1
  MainSwitch/1 -> S/C Conditioning/2(MainSwitch)
  Data Type Conversion/1 -> Multiport Switch/1
  SC/1 -> Multiport Switch/2
  Constant/1 -> Multiport Switch/3
  Multiport Switch/1 -> S/C Conditioning/1(SC)

== system MultipleAgentsChoice_NoVR/StatePropagation/SatelliteControlAccel/Agent Body1/Actual Thruster response/Ythruster1/Thruster1/ThrustBlock ==
  ForceRequest : Inport
  Short? : Inport  Port=2
  MainSwitch : Inport  Port=3
  Feed : Inport  Port=4
  CathodeEfficiency : Inport  Port=5
  ActiveThruster (logical) : Subsystem
  Bus Creator : BusCreator  Inputs=2
  Product : Product  RndMeth=Zero
  Product1 : Product  RndMeth=Zero
  Voltage/Current : Subsystem
  OutputForce : Outport
  ThrusterData : Outport  Port=2
  wires:
  MainSwitch/1 -> ActiveThruster (logical)/2(ThrusterOn?), Voltage/Current/2(MainSwitch)
  Short?/1 -> ActiveThruster (logical)/1(Short?), Voltage/Current/1(Short?)
  Feed/1 -> Voltage/Current/3(Feed?), ActiveThruster (logical)/3(Feed?)
  Voltage/Current/1(Voltage) -> Bus Creator/1  "voltage"
  Voltage/Current/2(Current) -> Bus Creator/2  "current"
  Bus Creator/1 -> ThrusterData/1
  ActiveThruster (logical)/1(Active) -> Product/1
  ForceRequest/1 -> [ForceRequest]
  CathodeEfficiency/1 -> [CathodeEfficiency]
  Product1/1 -> OutputForce/1
  [ForceRequest] -> Product/2
  Product/1 -> Product1/1
  [CathodeEfficiency] -> Product1/2

== system MultipleAgentsChoice_NoVR/StatePropagation/SatelliteControlAccel/Agent Body1/Actual Thruster response/Zthruster1/Thruster1/ForceShort ==
  note: Detect event and introduce short, otherwise pass through current result of short status
  Event : Inport
  SC : Inport  Port=2
  MainSwitch : Inport  Port=3
  Constant : Constant
  Data Type Conversion : DataTypeConversion
  Detect Increase : simulink/Logic and Bit Operations/Detect Increase  vinit=0  InputProcessing=Inherited  OutDataTypeStr=uint8
  Multiport Switch : MultiPortSwitch  DataPortOrder=Zero-based contiguous  Inputs=2  zeroidx=on
  S/C Conditioning : Subsystem
  SC_out : Outport
  wires:
  Multiport Switch/1 -> S/C Conditioning/1(SC)
  Constant/1 -> Multiport Switch/3
  SC/1 -> Multiport Switch/2
  Data Type Conversion/1 -> Multiport Switch/1
  MainSwitch/1 -> S/C Conditioning/2(MainSwitch)
  S/C Conditioning/1(Short?) -> SC_out/1
  Detect Increase/1 -> Data Type Conversion/1
  Event/1 -> Detect Increase/1

== system MultipleAgentsChoice_NoVR/StatePropagation/SatelliteControlAccel/Agent Body1/Actual Thruster response/Zthruster1/Thruster1/ThrustBlock ==
  ForceRequest : Inport
  Short? : Inport  Port=2
  MainSwitch : Inport  Port=3
  Feed : Inport  Port=4
  CathodeEfficiency : Inport  Port=5
  ActiveThruster (logical) : Subsystem
  Bus Creator : BusCreator  Inputs=2
  Product : Product  RndMeth=Zero
  Product1 : Product  RndMeth=Zero
  Voltage/Current : Subsystem
  OutputForce : Outport
  ThrusterData : Outport  Port=2
  wires:
  [CathodeEfficiency] -> Product1/2
  Product/1 -> Product1/1
  [ForceRequest] -> Product/2
  Product1/1 -> OutputForce/1
  CathodeEfficiency/1 -> [CathodeEfficiency]
  ForceRequest/1 -> [ForceRequest]
  ActiveThruster (logical)/1(Active) -> Product/1
  Bus Creator/1 -> ThrusterData/1
  Voltage/Current/2(Current) -> Bus Creator/2  "current"
  Voltage/Current/1(Voltage) -> Bus Creator/1  "voltage"
  Feed/1 -> ActiveThruster (logical)/3(Feed?), Voltage/Current/3(Feed?)
  Short?/1 -> Voltage/Current/1(Short?), ActiveThruster (logical)/1(Short?)
  MainSwitch/1 -> Voltage/Current/2(MainSwitch), ActiveThruster (logical)/2(ThrusterOn?)

== system MultipleAgentsChoice_NoVR/StatePropagation/SatelliteControlAccel/Agent Body2/Actual Thruster response/XYZthruster/Thruster1/ForceShort ==
  note: Detect event and introduce short, otherwise pass through current result of short status
  Event : Inport
  SC : Inport  Port=2
  MainSwitch : Inport  Port=3
  Constant : Constant
  Data Type Conversion : DataTypeConversion
  Detect Increase : simulink/Logic and Bit Operations/Detect Increase  vinit=0  InputProcessing=Inherited  OutDataTypeStr=uint8
  Multiport Switch : MultiPortSwitch  DataPortOrder=Zero-based contiguous  Inputs=2  zeroidx=on
  S/C Conditioning : Subsystem
  SC_out : Outport
  wires:
  Multiport Switch/1 -> S/C Conditioning/1(SC)
  Constant/1 -> Multiport Switch/3
  SC/1 -> Multiport Switch/2
  Data Type Conversion/1 -> Multiport Switch/1
  MainSwitch/1 -> S/C Conditioning/2(MainSwitch)
  S/C Conditioning/1(Short?) -> SC_out/1
  Detect Increase/1 -> Data Type Conversion/1
  Event/1 -> Detect Increase/1

== system MultipleAgentsChoice_NoVR/StatePropagation/SatelliteControlAccel/Agent Body2/Actual Thruster response/XYZthruster/Thruster1/ThrustBlock ==
  ForceRequest : Inport
  Short? : Inport  Port=2
  MainSwitch : Inport  Port=3
  Feed : Inport  Port=4
  CathodeEfficiency : Inport  Port=5
  ActiveThruster (logical) : Subsystem
  Bus Creator : BusCreator  Inputs=2
  Product : Product  RndMeth=Zero
  Product1 : Product  RndMeth=Zero
  Voltage/Current : Subsystem
  OutputForce : Outport
  ThrusterData : Outport  Port=2
  wires:
  [CathodeEfficiency] -> Product1/2
  Product/1 -> Product1/1
  [ForceRequest] -> Product/2
  CathodeEfficiency/1 -> [CathodeEfficiency]
  ForceRequest/1 -> [ForceRequest]
  ActiveThruster (logical)/1(Active) -> Product/1
  Bus Creator/1 -> ThrusterData/1
  Voltage/Current/2(Current) -> Bus Creator/2  "current"
  Voltage/Current/1(Voltage) -> Bus Creator/1  "voltage"
  Feed/1 -> ActiveThruster (logical)/3(Feed?), Voltage/Current/3(Feed?)
  Short?/1 -> Voltage/Current/1(Short?), ActiveThruster (logical)/1(Short?)
  MainSwitch/1 -> Voltage/Current/2(MainSwitch), ActiveThruster (logical)/2(ThrusterOn?)
  Product1/1 -> OutputForce/1

== system MultipleAgentsChoice_NoVR/StatePropagation/SatelliteControlAccel/Agent Body2/Actual Thruster response/Xthruster/Thruster1/ForceShort ==
  note: Detect event and introduce short, otherwise pass through current result of short status
  Event : Inport
  SC : Inport  Port=2
  MainSwitch : Inport  Port=3
  Constant : Constant
  Data Type Conversion : DataTypeConversion
  Detect Increase : simulink/Logic and Bit Operations/Detect Increase  vinit=0  InputProcessing=Inherited  OutDataTypeStr=uint8
  Multiport Switch : MultiPortSwitch  DataPortOrder=Zero-based contiguous  Inputs=2  zeroidx=on
  S/C Conditioning : Subsystem
  SC_out : Outport
  wires:
  Event/1 -> Detect Increase/1
  Detect Increase/1 -> Data Type Conversion/1
  S/C Conditioning/1(Short?) -> SC_out/1
  MainSwitch/1 -> S/C Conditioning/2(MainSwitch)
  Data Type Conversion/1 -> Multiport Switch/1
  SC/1 -> Multiport Switch/2
  Constant/1 -> Multiport Switch/3
  Multiport Switch/1 -> S/C Conditioning/1(SC)

== system MultipleAgentsChoice_NoVR/StatePropagation/SatelliteControlAccel/Agent Body2/Actual Thruster response/Xthruster/Thruster1/ThrustBlock ==
  ForceRequest : Inport
  Short? : Inport  Port=2
  MainSwitch : Inport  Port=3
  Feed : Inport  Port=4
  CathodeEfficiency : Inport  Port=5
  ActiveThruster (logical) : Subsystem
  Bus Creator : BusCreator  Inputs=2
  Product : Product  RndMeth=Zero
  Product1 : Product  RndMeth=Zero
  Voltage/Current : Subsystem
  OutputForce : Outport
  ThrusterData : Outport  Port=2
  wires:
  MainSwitch/1 -> ActiveThruster (logical)/2(ThrusterOn?), Voltage/Current/2(MainSwitch)
  Short?/1 -> ActiveThruster (logical)/1(Short?), Voltage/Current/1(Short?)
  Feed/1 -> Voltage/Current/3(Feed?), ActiveThruster (logical)/3(Feed?)
  Voltage/Current/1(Voltage) -> Bus Creator/1  "voltage"
  Voltage/Current/2(Current) -> Bus Creator/2  "current"
  Bus Creator/1 -> ThrusterData/1
  ActiveThruster (logical)/1(Active) -> Product/1
  ForceRequest/1 -> [ForceRequest]
  CathodeEfficiency/1 -> [CathodeEfficiency]
  [ForceRequest] -> Product/2
  Product/1 -> Product1/1
  [CathodeEfficiency] -> Product1/2
  Product1/1 -> OutputForce/1

== system MultipleAgentsChoice_NoVR/StatePropagation/SatelliteControlAccel/Agent Body2/Actual Thruster response/Ythruster1/Thruster1/ForceShort ==
  note: Detect event and introduce short, otherwise pass through current result of short status
  Event : Inport
  SC : Inport  Port=2
  MainSwitch : Inport  Port=3
  Constant : Constant
  Data Type Conversion : DataTypeConversion
  Detect Increase : simulink/Logic and Bit Operations/Detect Increase  vinit=0  InputProcessing=Inherited  OutDataTypeStr=uint8
  Multiport Switch : MultiPortSwitch  DataPortOrder=Zero-based contiguous  Inputs=2  zeroidx=on
  S/C Conditioning : Subsystem
  SC_out : Outport
  wires:
  Multiport Switch/1 -> S/C Conditioning/1(SC)
  Constant/1 -> Multiport Switch/3
  SC/1 -> Multiport Switch/2
  Data Type Conversion/1 -> Multiport Switch/1
  MainSwitch/1 -> S/C Conditioning/2(MainSwitch)
  S/C Conditioning/1(Short?) -> SC_out/1
  Detect Increase/1 -> Data Type Conversion/1
  Event/1 -> Detect Increase/1

== system MultipleAgentsChoice_NoVR/StatePropagation/SatelliteControlAccel/Agent Body2/Actual Thruster response/Ythruster1/Thruster1/ThrustBlock ==
  ForceRequest : Inport
  Short? : Inport  Port=2
  MainSwitch : Inport  Port=3
  Feed : Inport  Port=4
  CathodeEfficiency : Inport  Port=5
  ActiveThruster (logical) : Subsystem
  Bus Creator : BusCreator  Inputs=2
  Product : Product  RndMeth=Zero
  Product1 : Product  RndMeth=Zero
  Voltage/Current : Subsystem
  OutputForce : Outport
  ThrusterData : Outport  Port=2
  wires:
  [CathodeEfficiency] -> Product1/2
  Product/1 -> Product1/1
  [ForceRequest] -> Product/2
  CathodeEfficiency/1 -> [CathodeEfficiency]
  ForceRequest/1 -> [ForceRequest]
  ActiveThruster (logical)/1(Active) -> Product/1
  Bus Creator/1 -> ThrusterData/1
  Voltage/Current/2(Current) -> Bus Creator/2  "current"
  Voltage/Current/1(Voltage) -> Bus Creator/1  "voltage"
  Feed/1 -> ActiveThruster (logical)/3(Feed?), Voltage/Current/3(Feed?)
  Short?/1 -> Voltage/Current/1(Short?), ActiveThruster (logical)/1(Short?)
  MainSwitch/1 -> Voltage/Current/2(MainSwitch), ActiveThruster (logical)/2(ThrusterOn?)
  Product1/1 -> OutputForce/1

== system MultipleAgentsChoice_NoVR/StatePropagation/SatelliteControlAccel/Agent Body2/Actual Thruster response/Zthruster1/Thruster1/ForceShort ==
  note: Detect event and introduce short, otherwise pass through current result of short status
  Event : Inport
  SC : Inport  Port=2
  MainSwitch : Inport  Port=3
  Constant : Constant
  Data Type Conversion : DataTypeConversion
  Detect Increase : simulink/Logic and Bit Operations/Detect Increase  vinit=0  InputProcessing=Inherited  OutDataTypeStr=uint8
  Multiport Switch : MultiPortSwitch  DataPortOrder=Zero-based contiguous  Inputs=2  zeroidx=on
  S/C Conditioning : Subsystem
  SC_out : Outport
  wires:
  Event/1 -> Detect Increase/1
  Detect Increase/1 -> Data Type Conversion/1
  S/C Conditioning/1(Short?) -> SC_out/1
  MainSwitch/1 -> S/C Conditioning/2(MainSwitch)
  Data Type Conversion/1 -> Multiport Switch/1
  SC/1 -> Multiport Switch/2
  Constant/1 -> Multiport Switch/3
  Multiport Switch/1 -> S/C Conditioning/1(SC)

== system MultipleAgentsChoice_NoVR/StatePropagation/SatelliteControlAccel/Agent Body2/Actual Thruster response/Zthruster1/Thruster1/ThrustBlock ==
  ForceRequest : Inport
  Short? : Inport  Port=2
  MainSwitch : Inport  Port=3
  Feed : Inport  Port=4
  CathodeEfficiency : Inport  Port=5
  ActiveThruster (logical) : Subsystem
  Bus Creator : BusCreator  Inputs=2
  Product : Product  RndMeth=Zero
  Product1 : Product  RndMeth=Zero
  Voltage/Current : Subsystem
  OutputForce : Outport
  ThrusterData : Outport  Port=2
  wires:
  MainSwitch/1 -> ActiveThruster (logical)/2(ThrusterOn?), Voltage/Current/2(MainSwitch)
  Short?/1 -> ActiveThruster (logical)/1(Short?), Voltage/Current/1(Short?)
  Feed/1 -> Voltage/Current/3(Feed?), ActiveThruster (logical)/3(Feed?)
  Voltage/Current/1(Voltage) -> Bus Creator/1  "voltage"
  Voltage/Current/2(Current) -> Bus Creator/2  "current"
  Bus Creator/1 -> ThrusterData/1
  ActiveThruster (logical)/1(Active) -> Product/1
  ForceRequest/1 -> [ForceRequest]
  CathodeEfficiency/1 -> [CathodeEfficiency]
  [ForceRequest] -> Product/2
  Product/1 -> Product1/1
  [CathodeEfficiency] -> Product1/2
  Product1/1 -> OutputForce/1

== system MultipleAgentsChoice_NoVR/StatePropagation/SatelliteControlAccel/Agent Body3/Actual Thruster response/XYZthruster/Thruster1/ForceShort ==
  note: Detect event and introduce short, otherwise pass through current result of short status
  Event : Inport
  SC : Inport  Port=2
  MainSwitch : Inport  Port=3
  Constant : Constant
  Data Type Conversion : DataTypeConversion
  Detect Increase : simulink/Logic and Bit Operations/Detect Increase  vinit=0  InputProcessing=Inherited  OutDataTypeStr=uint8
  Multiport Switch : MultiPortSwitch  DataPortOrder=Zero-based contiguous  Inputs=2  zeroidx=on
  S/C Conditioning : Subsystem
  SC_out : Outport
  wires:
  Multiport Switch/1 -> S/C Conditioning/1(SC)
  Constant/1 -> Multiport Switch/3
  SC/1 -> Multiport Switch/2
  Data Type Conversion/1 -> Multiport Switch/1
  MainSwitch/1 -> S/C Conditioning/2(MainSwitch)
  S/C Conditioning/1(Short?) -> SC_out/1
  Detect Increase/1 -> Data Type Conversion/1
  Event/1 -> Detect Increase/1

== system MultipleAgentsChoice_NoVR/StatePropagation/SatelliteControlAccel/Agent Body3/Actual Thruster response/XYZthruster/Thruster1/ThrustBlock ==
  ForceRequest : Inport
  Short? : Inport  Port=2
  MainSwitch : Inport  Port=3
  Feed : Inport  Port=4
  CathodeEfficiency : Inport  Port=5
  ActiveThruster (logical) : Subsystem
  Bus Creator : BusCreator  Inputs=2
  Product : Product  RndMeth=Zero
  Product1 : Product  RndMeth=Zero
  Voltage/Current : Subsystem
  OutputForce : Outport
  ThrusterData : Outport  Port=2
  wires:
  [CathodeEfficiency] -> Product1/2
  Product/1 -> Product1/1
  [ForceRequest] -> Product/2
  CathodeEfficiency/1 -> [CathodeEfficiency]
  ForceRequest/1 -> [ForceRequest]
  ActiveThruster (logical)/1(Active) -> Product/1
  Bus Creator/1 -> ThrusterData/1
  Voltage/Current/2(Current) -> Bus Creator/2  "current"
  Voltage/Current/1(Voltage) -> Bus Creator/1  "voltage"
  Feed/1 -> ActiveThruster (logical)/3(Feed?), Voltage/Current/3(Feed?)
  Short?/1 -> Voltage/Current/1(Short?), ActiveThruster (logical)/1(Short?)
  MainSwitch/1 -> Voltage/Current/2(MainSwitch), ActiveThruster (logical)/2(ThrusterOn?)
  Product1/1 -> OutputForce/1

== system MultipleAgentsChoice_NoVR/StatePropagation/SatelliteControlAccel/Agent Body3/Actual Thruster response/Xthruster/Thruster1/ForceShort ==
  note: Detect event and introduce short, otherwise pass through current result of short status
  Event : Inport
  SC : Inport  Port=2
  MainSwitch : Inport  Port=3
  Constant : Constant
  Data Type Conversion : DataTypeConversion
  Detect Increase : simulink/Logic and Bit Operations/Detect Increase  vinit=0  InputProcessing=Inherited  OutDataTypeStr=uint8
  Multiport Switch : MultiPortSwitch  DataPortOrder=Zero-based contiguous  Inputs=2  zeroidx=on
  S/C Conditioning : Subsystem
  SC_out : Outport
  wires:
  Event/1 -> Detect Increase/1
  Detect Increase/1 -> Data Type Conversion/1
  S/C Conditioning/1(Short?) -> SC_out/1
  MainSwitch/1 -> S/C Conditioning/2(MainSwitch)
  Data Type Conversion/1 -> Multiport Switch/1
  SC/1 -> Multiport Switch/2
  Constant/1 -> Multiport Switch/3
  Multiport Switch/1 -> S/C Conditioning/1(SC)

== system MultipleAgentsChoice_NoVR/StatePropagation/SatelliteControlAccel/Agent Body3/Actual Thruster response/Xthruster/Thruster1/ThrustBlock ==
  ForceRequest : Inport
  Short? : Inport  Port=2
  MainSwitch : Inport  Port=3
  Feed : Inport  Port=4
  CathodeEfficiency : Inport  Port=5
  ActiveThruster (logical) : Subsystem
  Bus Creator : BusCreator  Inputs=2
  Product : Product  RndMeth=Zero
  Product1 : Product  RndMeth=Zero
  Voltage/Current : Subsystem
  OutputForce : Outport
  ThrusterData : Outport  Port=2
  wires:
  MainSwitch/1 -> ActiveThruster (logical)/2(ThrusterOn?), Voltage/Current/2(MainSwitch)
  Short?/1 -> ActiveThruster (logical)/1(Short?), Voltage/Current/1(Short?)
  Feed/1 -> Voltage/Current/3(Feed?), ActiveThruster (logical)/3(Feed?)
  Voltage/Current/1(Voltage) -> Bus Creator/1  "voltage"
  Voltage/Current/2(Current) -> Bus Creator/2  "current"
  Bus Creator/1 -> ThrusterData/1
  ActiveThruster (logical)/1(Active) -> Product/1
  ForceRequest/1 -> [ForceRequest]
  CathodeEfficiency/1 -> [CathodeEfficiency]
  [ForceRequest] -> Product/2
  Product/1 -> Product1/1
  [CathodeEfficiency] -> Product1/2
  Product1/1 -> OutputForce/1

== system MultipleAgentsChoice_NoVR/StatePropagation/SatelliteControlAccel/Agent Body3/Actual Thruster response/Ythruster1/Thruster1/ForceShort ==
  note: Detect event and introduce short, otherwise pass through current result of short status
  Event : Inport
  SC : Inport  Port=2
  MainSwitch : Inport  Port=3
  Constant : Constant
  Data Type Conversion : DataTypeConversion
  Detect Increase : simulink/Logic and Bit Operations/Detect Increase  vinit=0  InputProcessing=Inherited  OutDataTypeStr=uint8
  Multiport Switch : MultiPortSwitch  DataPortOrder=Zero-based contiguous  Inputs=2  zeroidx=on
  S/C Conditioning : Subsystem
  SC_out : Outport
  wires:
  Multiport Switch/1 -> S/C Conditioning/1(SC)
  Constant/1 -> Multiport Switch/3
  SC/1 -> Multiport Switch/2
  Data Type Conversion/1 -> Multiport Switch/1
  MainSwitch/1 -> S/C Conditioning/2(MainSwitch)
  S/C Conditioning/1(Short?) -> SC_out/1
  Detect Increase/1 -> Data Type Conversion/1
  Event/1 -> Detect Increase/1
